simulink model "CarClosedLoopPositionControl"  (R2019a)
settings: Solver=VariableStepAuto  StartTime=0.0  StopTime=30.0  FixedStep=0.01  RelTol=1e-4
libraries: simulink x6
settings Model: Creator=janni  LastModifiedBy=janni

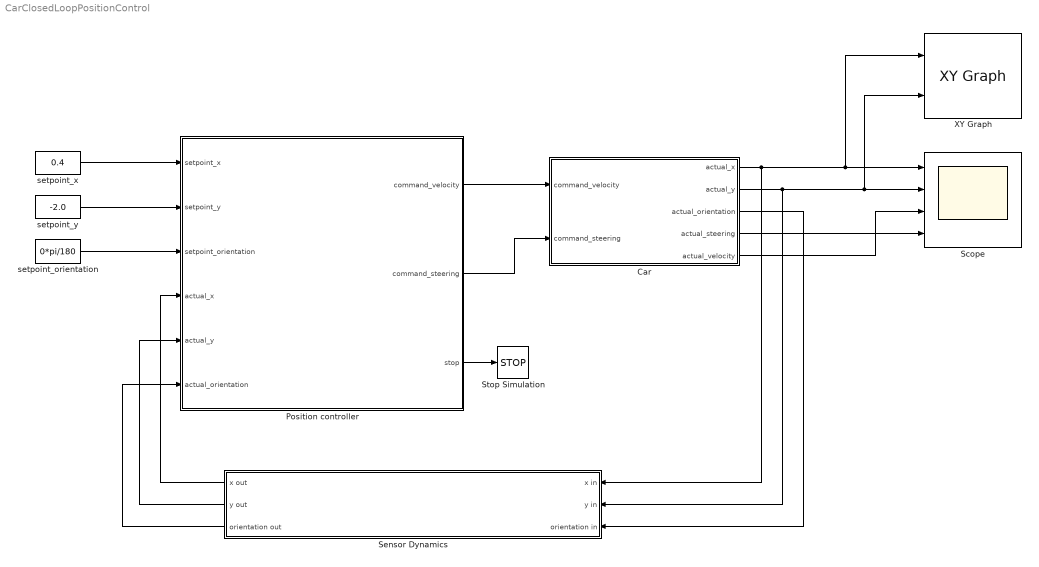
== system CarClosedLoopPositionControl ==
  Car : Subsystem
  Position controller : Subsystem
  Scope : Scope  NumInputPorts=4
  Sensor Dynamics : Subsystem
  Stop Simulation : Stop
  XY Graph : simulink/Sinks/XY Graph  xmin=-3  xmax=3  ymin=-3  ymax=3  st=-1
  setpoint_orientation : Constant  Value=0*pi/180
  setpoint_x : Constant  Value=0.4
  setpoint_y : Constant  Value=-2.0
  wires:
  setpoint_x/1 -> Position controller/1(setpoint_x)
  Car/1(actual_x) -> Sensor Dynamics/1(x in), XY Graph/1, Scope/1
  Car/2(actual_y) -> Sensor Dynamics/2(y in), XY Graph/2, Scope/2
  setpoint_y/1 -> Position controller/2(setpoint_y)
  Car/3(actual_orientation) -> Sensor Dynamics/3(orientation in)
  setpoint_orientation/1 -> Position controller/3(setpoint_orientation)
  Position controller/1(command_velocity) -> Car/1(command_velocity)
  Position controller/2(command_steering) -> Car/2(command_steering)
  Position controller/3(stop) -> Stop Simulation/1
  Sensor Dynamics/1(x out) -> Position controller/4(actual_x)
  Sensor Dynamics/2(y out) -> Position controller/5(actual_y)
  Sensor Dynamics/3(orientation out) -> Position controller/6(actual_orientation)
  Car/4(actual_steering) -> Scope/4
  Car/5(actual_velocity) -> Scope/3

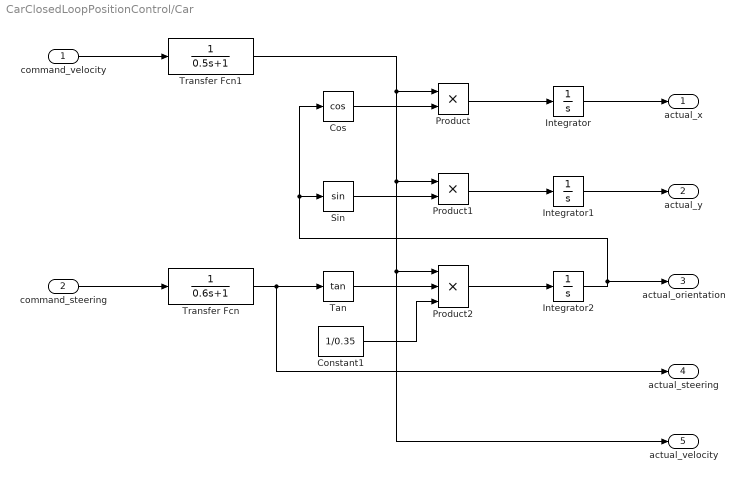
== system CarClosedLoopPositionControl/Car ==
  command_velocity : Inport
  command_steering : Inport  Port=2
  Constant1 : Constant  Value=1/0.35
  Cos : Trigonometry  Operator=cos
  Integrator : Integrator
  Integrator1 : Integrator
  Integrator2 : Integrator
  Product : Product
  Product1 : Product
  Product2 : Product  Inputs=3
  Sin : Trigonometry
  Tan : Trigonometry  Operator=tan
  Transfer Fcn : TransferFcn  Denominator=[0.6 1]
  Transfer Fcn1 : TransferFcn  Denominator=[0.5 1]
  actual_x : Outport
  actual_y : Outport  Port=2
  actual_orientation : Outport  Port=3
  actual_steering : Outport  Port=4
  actual_velocity : Outport  Port=5
  wires:
  Product/1 -> Integrator/1
  Cos/1 -> Product/2
  Tan/1 -> Product2/2
  Product2/1 -> Integrator2/1
  Product1/1 -> Integrator1/1
  Constant1/1 -> Product2/3
  Integrator2/1 -> actual_orientation/1, Cos/1, Sin/1
  command_velocity/1 -> Transfer Fcn1/1
  Sin/1 -> Product1/2
  command_steering/1 -> Transfer Fcn/1
  Integrator/1 -> actual_x/1
  Integrator1/1 -> actual_y/1
  Transfer Fcn/1 -> actual_steering/1, Tan/1
  Transfer Fcn1/1 -> Product/1, Product1/1, Product2/1, actual_velocity/1

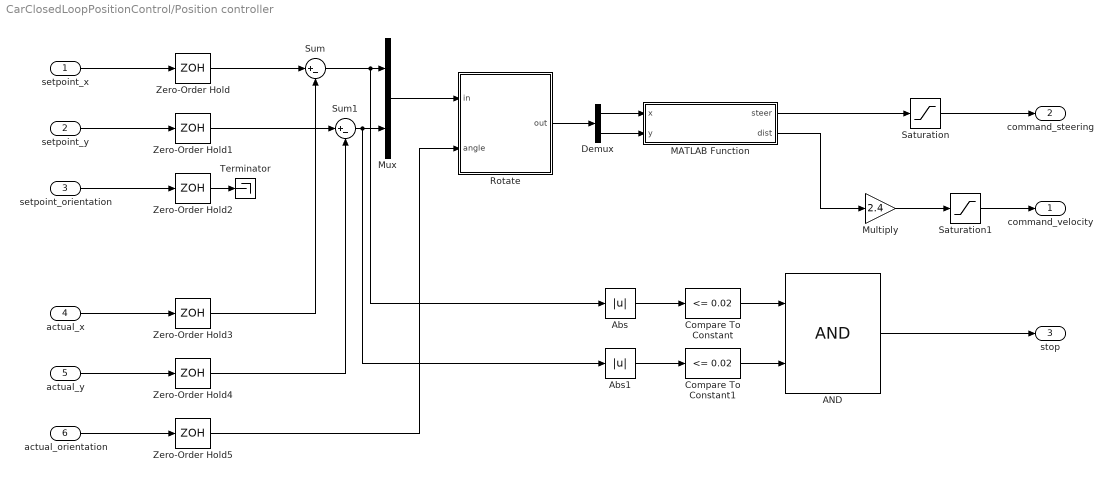
== system CarClosedLoopPositionControl/Position controller ==
  setpoint_x : Inport
  setpoint_y : Inport  Port=2
  setpoint_orientation : Inport  Port=3
  actual_x : Inport  Port=4
  actual_y : Inport  Port=5
  actual_orientation : Inport  Port=6
  AND : Logic  AllPortsSameDT=off  OutDataTypeStr=boolean
  Abs : Abs
  Abs1 : Abs
  Compare To Constant : simulink/Logic and Bit Operations/Compare To Constant  relop=<=  const=0.02  OutDataTypeStr=boolean
  Compare To Constant1 : simulink/Logic and Bit Operations/Compare To Constant  relop=<=  const=0.02  OutDataTypeStr=boolean
  Demux : Demux  Outputs=2
  MATLAB Function : MATLAB Function  TreatAsAtomicUnit=on
  Multiply : Gain  Gain=2.4
  Mux : Mux  Inputs=2
  Rotate : Subsystem
  Saturation : Saturate  UpperLimit=pi/4  LowerLimit=-pi/4
  Saturation1 : Saturate  UpperLimit=1.2  LowerLimit=-1.2
  Sum : Sum  Inputs=|+-
  Sum1 : Sum  Inputs=|+-
  Terminator : Terminator
  Zero-Order Hold{,1..5} (6 alike) : ZeroOrderHold  SampleTime=0.01
  command_velocity : Outport
  command_steering : Outport  Port=2
  stop : Outport  Port=3
  wires:
  setpoint_x/1 -> Zero-Order Hold/1
  setpoint_y/1 -> Zero-Order Hold1/1
  setpoint_orientation/1 -> Zero-Order Hold2/1
  actual_y/1 -> Zero-Order Hold4/1
  actual_x/1 -> Zero-Order Hold3/1
  actual_orientation/1 -> Zero-Order Hold5/1
  Rotate/1(out) -> Demux/1
  Demux/1 -> MATLAB Function/1(x)
  Demux/2 -> MATLAB Function/2(y)
  MATLAB Function/1(steer) -> Saturation/1
  MATLAB Function/2(dist) -> Multiply/1
  Saturation/1 -> command_steering/1
  Abs/1 -> Compare To Constant/1
  Zero-Order Hold1/1 -> Sum1/1
  Zero-Order Hold/1 -> Sum/1
  Zero-Order Hold2/1 -> Terminator/1
  Zero-Order Hold3/1 -> Sum/2
  Zero-Order Hold4/1 -> Sum1/2
  Zero-Order Hold5/1 -> Rotate/2(angle)
  Sum/1 -> Abs/1, Mux/1
  Mux/1 -> Rotate/1(in)
  Sum1/1 -> Abs1/1, Mux/2
  Abs1/1 -> Compare To Constant1/1
  Compare To Constant/1 -> AND/1
  Compare To Constant1/1 -> AND/2
  AND/1 -> stop/1
  Multiply/1 -> Saturation1/1
  Saturation1/1 -> command_velocity/1

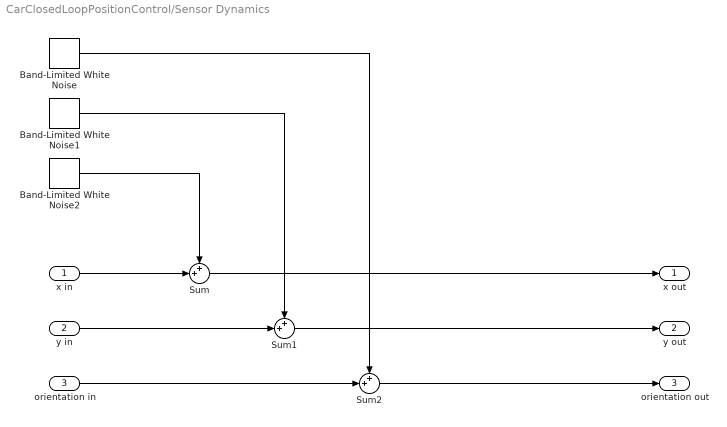
== system CarClosedLoopPositionControl/Sensor Dynamics ==
  x in : Inport
  y in : Inport  Port=2
  orientation in : Inport  Port=3
  Band-Limited White Noise : simulink/Sources/Band-Limited White Noise  Cov=0.0002  Ts=0.01  seed=[62354]
  Band-Limited White Noise1 : simulink/Sources/Band-Limited White Noise  Cov=0.0002  Ts=0.01  seed=[46711]
  Band-Limited White Noise2 : simulink/Sources/Band-Limited White Noise  Cov=0.0002  Ts=0.01  seed=[23341]
  Sum : Sum  Inputs=++|
  Sum1 : Sum  Inputs=++|
  Sum2 : Sum  Inputs=++|
  x out : Outport
  y out : Outport  Port=2
  orientation out : Outport  Port=3
  wires:
  x in/1 -> Sum/2
  y in/1 -> Sum1/2
  orientation in/1 -> Sum2/2
  Sum2/1 -> orientation out/1
  Sum1/1 -> y out/1
  Sum/1 -> x out/1
  Band-Limited White Noise2/1 -> Sum/1
  Band-Limited White Noise1/1 -> Sum1/1
  Band-Limited White Noise/1 -> Sum2/1

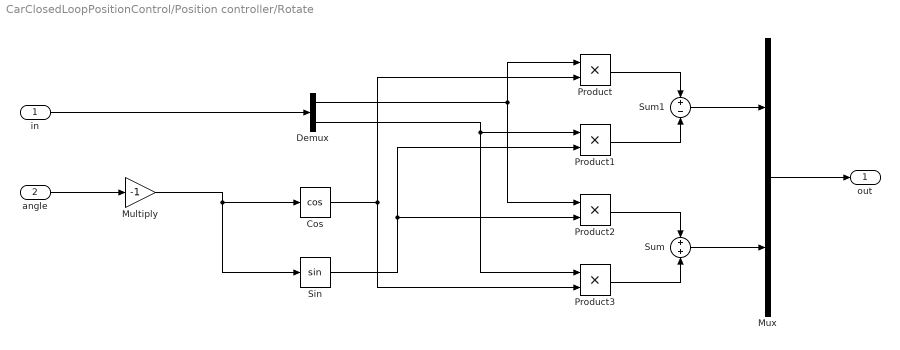
== system CarClosedLoopPositionControl/Position controller/Rotate ==
  in : Inport
  angle : Inport  Port=2
  Cos : Trigonometry  Operator=cos
  Demux : Demux  Outputs=2
  Multiply : Gain  Gain=-1
  Mux : Mux  Inputs=2
  Product{,1..3} (4 alike) : Product
  Sin : Trigonometry
  Sum : Sum  Inputs=+|+
  Sum1 : Sum  Inputs=+|-
  out : Outport
  wires:
  in/1 -> Demux/1
  Product/1 -> Sum1/1
  Product1/1 -> Sum1/2
  Product2/1 -> Sum/1
  Product3/1 -> Sum/2
  Sum/1 -> Mux/2
  Sum1/1 -> Mux/1
  Mux/1 -> out/1
  angle/1 -> Multiply/1
  Cos/1 -> Product/2, Product3/2
  Sin/1 -> Product2/2, Product1/2
  Demux/1 -> Product2/1, Product/1
  Demux/2 -> Product3/1, Product1/1
  Multiply/1 -> Sin/1, Cos/1

== matlab function CarClosedLoopPositionControl/Position controller/MATLAB Function ==
  data: x input; steer output; y input; dist output
function [steer, dist]= plan_circle(x, y)

l = 0.34;

if abs(x) > 0.01
    if y < 0
        r = (y^2 + x^2) / (2 * -y);
        phi = asin(x / r);

        if 2 * r < l
            r = l / 2;
        end
        
        steer = -2 * asin(l / (2 * r));
        dist = r * phi;
    elseif y > 0
        r = (y^2 + x^2) / (2 * y);
        phi = asin(x / r);
        
        if 2 * r < l
            r = l / 2;
        end

        steer = 2 * asin(l / (2 * r));
        dist = r * phi;
    else
        steer = 0;
        dist = x;
    end
else
    steer = 0.0;
    dist = 0.0;
end
